simulink model "week1_problem6"  (R2020b)
settings: Solver=VariableStepAuto  StartTime=0.0  StopTime=10.0  RelTol=1e-3
libraries: dspsrcs4 x1
settings Model: Creator=gauri  LastModifiedBy=mluser

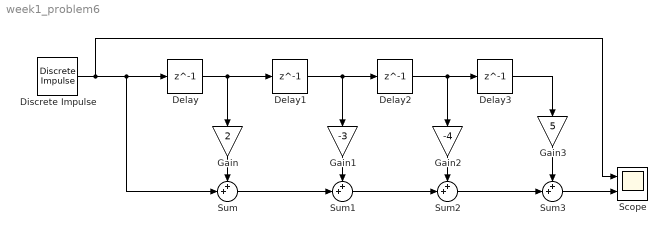
== system week1_problem6 ==
  Delay{,1..3} (4 alike) : Delay  DelayLength=1  InitialCondition=0
  Discrete Impulse : dspsrcs4/Discrete  Impulse  Delay=0  SampleTime=1  FrameSample=1  OutputFrames=off  dataType=double  isSigned=on  wordLen=16  udDataType=sfix(16)  fracBitsMode=Best precision  numFracBits=15  OutDataTypeStr=double  LastOutDataTypeStr=double
  Gain : Gain  Gain=2
  Gain1 : Gain  Gain=-3
  Gain2 : Gain  Gain=-4
  Gain3 : Gain  Gain=5
  Scope : Scope  NumInputPorts=2
  Sum{,1..3} (4 alike) : Sum  Inputs=++|
  wires:
  Discrete Impulse/1 -> Scope/1, Sum/2, Delay/1
  Delay/1 -> Gain/1, Delay1/1
  Delay1/1 -> Gain1/1, Delay2/1
  Delay2/1 -> Gain2/1, Delay3/1
  Gain/1 -> Sum/1
  Gain1/1 -> Sum1/1
  Sum/1 -> Sum1/2
  Gain2/1 -> Sum2/1
  Sum1/1 -> Sum2/2
  Delay3/1 -> Gain3/1
  Gain3/1 -> Sum3/1
  Sum2/1 -> Sum3/2
  Sum3/1 -> Scope/2
